simulink model "mat_jobfnet2"  (R2024a)
settings: Solver=VariableStepAuto  StartTime=0.0  StopTime=100  RelTol=1e-3
values from neighbouring files (symbols this model uses):
  A = 2.2    [sim_jobfnet2.m]
  Cd = 0.3    [sim_jobfnet2.m]
  Cr = 0.015    [sim_jobfnet2.m]
  g = 9.81    [sim_jobfnet2.m]
  m = 1500    [sim_jobfnet2.m]
  r_gear = 4    [sim_jobfnet2.m]
  r_wheel = 0.3    [sim_jobfnet2.m]
  rho = 1.225    [sim_jobfnet2.m]
  tm = 21000    [sim_jobfnet2.m]
settings Model: Creator=Akshata  LastModifiedBy=Akshata

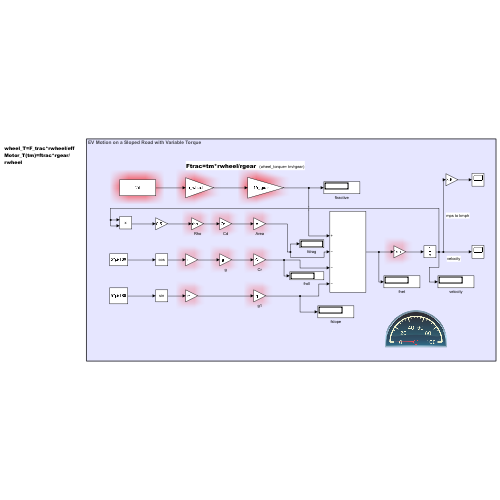
[thumbnail: Simulink's stored preview of the top-level diagram]
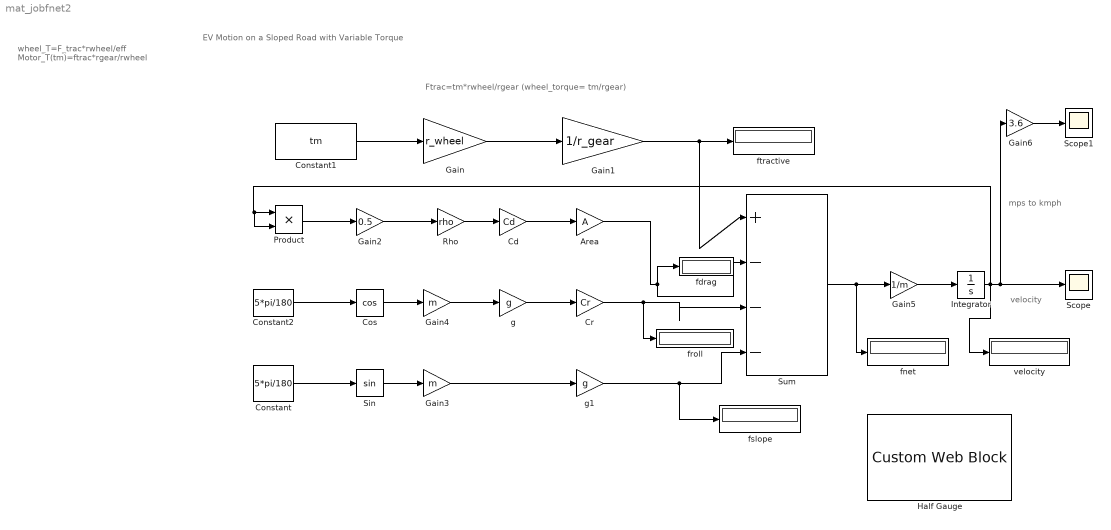
== system mat_jobfnet2 ==
  note: Ftrac=tm*rwheel/rgear (wheel_torque= tm/rgear)
  note: velocity
  note: mps to kmph
  note: EV Motion on a Sloped Road with Variable Torque
  note: wheel_T=F_trac*rwheel/eff
      | Motor_T(tm)=ftrac*rgear/rwheel
  Area : Gain  Gain=A
  Cd : Gain  Gain=Cd
  Constant : Constant  Value=5*pi/180
  Constant1 : Constant  Value=tm
  Constant2 : Constant  Value=5*pi/180
  Cos : Trigonometry  Operator=cos
  Cr : Gain  Gain=Cr
  Gain : Gain  Gain=r_wheel
  Gain1 : Gain  Gain=1/r_gear
  Gain2 : Gain  Gain=0.5
  Gain3 : Gain  Gain=m
  Gain4 : Gain  Gain=m
  Gain5 : Gain  Gain=1/m
  Gain6 : Gain  Gain=3.6
  Half Gauge : CustomWebBlock  LabelPosition=Hide  ShowInitialText=on  Configuration="{\"components\":[{\"name\":\"CircularScaleComponent\",\"settings\":{\"bounds\":{\"max\":100,\"min\":0,\"tickInterval\":\"auto\"},\"direction\":\"cw\",\"flipLimits\":0,\"innerRadius\":0.75,\"internalTickHeightScaleFactor\":1,\"labelColor\":[255,255,200],\"labelFont\":{\"font\":\"Arial\",\"fontSize\":12},\"labelRadius\":0.528,\"labelTransparency\":1,\"minorTickHeightScaleFactor\":0.2,\"needleImage\":{\"size\":[200,50],\"src\":\"data:image\\/svg+xml;base64,PD94bWwgdmVyc2lvbj0iMS4wIiBlbmNvZGluZz0idXRmLTgiPz4KPCEtLSBHZW5lcmF0b3I6IEFkb2JlIElsbHVzdHJhdG9yIDI0LjEuMiwgU1ZHIEV4cG9ydCBQbHVnLUluIC4gU1ZHIFZlcnNpb246IDYuMDAgQnVpbGQgMCkgIC0tPgo8c3ZnIHZlcnNpb249IjEuMSIgaWQ9IkxheWVyXzEiIHhtbG5zPSJodHRwOi8vd3d3LnczLm9yZy8yMDAwL3N2ZyIgeG1sbnM6eGxpbms9Imh0dHA6Ly93d3cudzMub3JnLzE5OTkveGxpbmsiIHg9IjBweCIgeT0iMHB4IgoJIHZpZXdCb3g9IjAgMCAyMDAgNTAiIHN0eWxlPSJlbmFibGUtYmFja2dyb3VuZDpuZXcgMCAwIDIwMCA1MDsiIHhtbDpzcGFjZT0icHJlc2VydmUiPgo8c3R5bGUgdHlwZT0idGV4dC9jc3MiPgoJLnN0MHtmaWxsOiNFQzIxMjc7fQo8L3N0eWxlPgo8cGF0aCBjbGFzcz0ic3QwIiBkPSJNMTYyLjgsMTMuN0MxNjksNC40LDE4MS43LDEuOSwxOTEsOC4xczExLjgsMTguOSw1LjYsMjguMnMtMTguOSwxMS44LTI4LjIsNS42bDAsMAoJQzE1OS4xLDM1LjYsMTU2LjYsMjMsMTYyLjgsMTMuN0wxNjIuOCwxMy43eiBNMTY1LjgsMTUuOGMtNS4xLDcuNi0zLjEsMTcuOSw0LjYsMjNjNy42LDUuMSwxNy45LDMuMSwyMy00LjYKCWM1LjEtNy42LDMuMS0xNy45LTQuNi0yM2wwLDBDMTgxLjIsNi4yLDE3MC45LDguMiwxNjUuOCwxNS44eiIvPgo8cGF0aCBjbGFzcz0ic3QwIiBkPSJNMC40LDI1Ljl2LTMuM2wxNTktMi41Yy0wLjcsMi42LTAuNyw1LjIsMCw3LjhMMC40LDI1Ljl6Ii8+CjxjaXJjbGUgY2xhc3M9InN0MCIgY3g9IjE3OS42IiBjeT0iMjQiIHI9IjAuNyIvPgo8L3N2Zz4K\"},\"needleOffset\":[0.18464878250906522,0],\"needleOrientation\":-45,\"needleRotation\":180,\"needleSize\":{\"height\":0.11741692305346914,\"width\":0.46108337545091255},\"outerRadius\":0.9,\"position\":[0.05,0.05,0.9,1.6],\"referencePoint\":\"auto\",\"scaleAngle\":180,\"scaleAngleOffset\":180,\"scaleColors\":[],\"scaleColorsSize\":0.2,\"scaleDirection\":\"CW\",\"scalePosition\":[0,0,1,1],\"showLabels\":1,\"showMinorTicks\":1,\"showSpanLine\":1,\"showTicks\":1,\"tickColor\":[252,252,197],\"tickTransparency\":1,\"valueBarColor\":[0,114,189],\"valueBarPosition\":[0,0,1,1],\"valueBarSize\":0.2,\"valueBarTransparency\":1}},{\"name\":\"BackgroundImageComponent\",\"settings\":{\"image\":{\"size\":[252,150],\"src\":\"data:image\\/svg+xml;base64,PD94bWwgdmVyc2lvbj0iMS4wIiBlbmNvZGluZz0idXRmLTgiPz4KPCEtLSBHZW5lcmF0b3I6IEFkb2JlIElsbHVzdHJhdG9yIDI2LjEuMCwgU1ZHIEV4cG9ydCBQbHVnLUluIC4gU1ZHIFZlcnNpb246IDYuMDAgQnVpbGQgMCkgIC0tPgo8c3ZnIHZlcnNpb249IjEuMSIKCSBpZD0iTGF5ZXJfMl8xXyIgeG1sbnM6Y2M9Imh0dHA6Ly9jcmVhdGl2ZWNvbW1vbnMub3JnL25zIyIgeG1sbnM6ZGM9Imh0dHA6Ly9wdXJsLm9yZy9kYy9lbGVtZW50cy8xLjEvIiB4bWxuczppbmtzY2FwZT0iaHR0cDovL3d3dy5pbmtzY2FwZS5vcmcvbmFt ...(+5492 chars)\",\"srcOrientation\":\"Right\"},\"position\":[0,0,1,1],\"scaleMode\":\"0\"}},{\"name\":\"ForegroundImageComponent\",\"settings\":{\"image\":{\"size\":[0,0],\"src\":\"default\",\"srcOrientation\":[]},\"isForeground\":1,\"position\":[0,0,1,1],\"scaleMode\":\"0\"}}],\"settings\":{\"BindingType\":\"signal\",\"aspectRatio\":1.032258064516129,\"backgroundColor\":[0,0,0,\"1\"],\"backgroundOffset\":1,\"backgroundOpacity\":1,\"direction\":\"cw\",\"fixedAspectRatio\":\"on\",\"flipLimits\":0,\"orientation\":\"horizontal\",\"showBackgroundColor\":false,\"value\":0,\"variant\":\"half\",\"version\":\"R2023a\"},\"type\":\"CircularGauge\"}"
  Integrator : Integrator
  Product : Product
  Rho : Gain  Gain=rho
  Scope : Scope
  Scope1 : Scope
  Sin : Trigonometry
  Sum : Sum  Inputs=|+---
  fdrag : Display
  fnet : Display
  froll : Display
  fslope : Display
  ftractive : Display
  g : Gain  Gain=g
  g1 : Gain  Gain=g
  velocity : Display
  wires:
  Product/1 -> Gain2/1
  Gain2/1 -> Rho/1
  Cd/1 -> Area/1
  Gain4/1 -> g/1
  Rho/1 -> Cd/1
  g/1 -> Cr/1
  Gain3/1 -> g1/1
  Constant/1 -> Sin/1
  Sin/1 -> Gain3/1
  Cos/1 -> Gain4/1
  Constant2/1 -> Cos/1
  Constant1/1 -> Gain/1
  Gain/1 -> Gain1/1
  Gain1/1 -> ftractive/1, Sum/1
  Area/1 -> fdrag/1, Sum/2
  Cr/1 -> froll/1, Sum/3
  g1/1 -> Sum/4, fslope/1
  Sum/1 -> fnet/1, Gain5/1
  Gain5/1 -> Integrator/1
  Integrator/1 -> Scope/1, Gain6/1, velocity/1, Product/2, Product/1
  Gain6/1 -> Scope1/1
